simulink model "vehicleModelMotor"  (R2024b)
settings: Solver=VariableStepAuto  StartTime=0.0  StopTime=1200  MaxStep=0.1  RelTol=1e-3  AbsTol=1e-3
PreLoadFcn:
  | setVehicleParam
undefined symbols (not defined in the file): wheelInertia
libraries: fl_lib x8, sdl_lib x8, nesl_utility x5, ee_lib x3
settings Model: Creator=lnicolet  LastModifiedBy=lnicolet
settings SolverCC: AutoScaleAbsTol=off  AlgebraicLoopSolver=TrustRegion  MaxZcPerStep=1
settings DebuggingCC: UnconnectedInputMsg=warning  UnconnectedOutputMsg=warning  UnconnectedLineMsg=warning  SymbolicDimsDataTypeCodeGenerationDiagnostic=none
settings ModelReferenceCC: EnableRefExpFcnMdlSchedulingChecks=on
settings SFSimCC: CustomCodeUndefinedFunction=UseInterfaceOnly
settings RTWCC: GPUComputeCapability=3.5  DLArmComputeVersion=19.05
settings SimscapeCC: SimscapeLogType=all  SimscapeLogSimulationStatistics=on  SimscapeLogLimitData=off  SimscapeLogDataHistory=10000

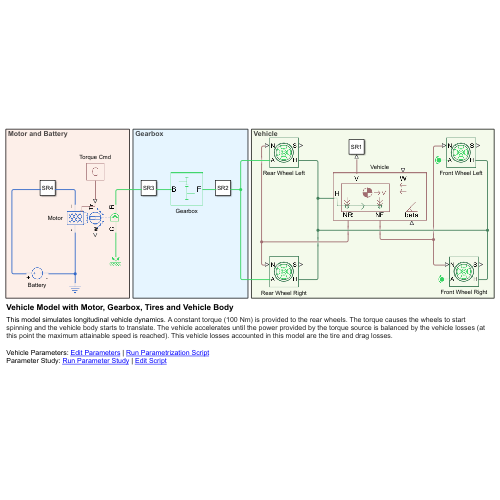
[thumbnail: Simulink's stored preview of the top-level diagram]
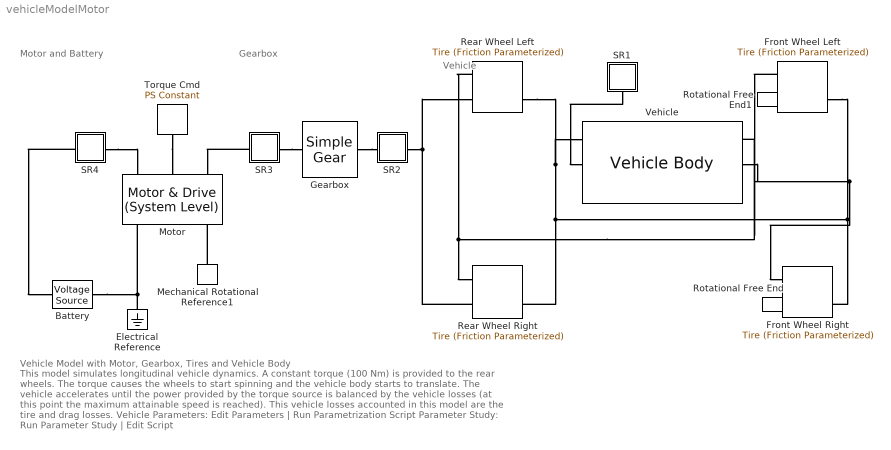
== system vehicleModelMotor ==
  note: Vehicle
  note: Gearbox
  note: This model simulates longitudinal vehicle dynamics. A constant torque (100 Nm) is provided to the rear wheels. The torque causes the wheels to start spinning and the vehicle body starts to translate. The vehicle accelerates until the power provided by the torque source is balanced by the vehicle losses (at this point the maximum attainable speed is reached). This vehicle losses accounted in this model are the tire and drag losses.
      |
      | Vehicle Parameters: Edit Parameters | Run Parametrization Script
      | Parameter Study: Run Parameter Study | Edit Script
  note: Vehicle Model with Motor, Gearbox, Tires and Vehicle Body
  note: Motor and Battery
  Battery : ee_lib/Sources/Voltage Source  dc_voltage=300 V  ac_voltage=0 V  ac_shift=0 rad  ac_frequency=60 Hz  noise_mode=ee.enum.sources.noise.Disabled  PSD=0 V^2/Hz  sample_time=1e-3 s  repeatability=ee.enum.sources.repeatability.NotRepeatable  user_seed=0  auto_seed=545404223  i_specify=off  i_priority=None  i=0 A  i_nominal_specify=off  i_nominal_value=1  i_nominal_unit=A  v_specify=off  v_priority=None  v=0 V  v_nominal_specify=off  v_nominal_value=1  v_nominal_unit=V
  Electrical Reference : fl_lib/Electrical/Electrical Elements/Electrical Reference
  Front Wheel Left : sdl_lib/Tires & Vehicles/Tire (Friction Parameterized)  r_tire=wheelRadius m  slip_output=sdl.enum.SlipOutput.Relative  friction_model=sdl.enum.friction_model_var.fixed  mu_static=0.90  mu_kinetic=0.70  slip_vector=[-1, .6, .15, .06, .02, 0] rad/s  mu_kinetic_vector=[.7, .7, .75, .8, .88, .89]  interp_method=simscape.enum.interpolation.linear  extrap_method=simscape.enum.extrapolation.linear  model_compliance=sdl.enum.compliance.off  stiffness=1e6 N/m  damping=1000 N*s/m  model_inertia=true  wheel_inertia=wheelInertia(1) kg*m^2  belt_inertia=wheelInertia(2) kg*m^2  initial_velocity=wheelSpeedStart rad/s  model_resistance=simscape.enum.onoff.on  resistance_model=sdl.enum.RollingResistance.Constant  coeff=0.015  p_tire=250e3 Pa  alpha=-0.003  beta=0.97  coeff_a=84e-4  coeff_b=6.2e-4 s/m  coeff_c=1.6e-4 s^2/m^2  v_thr=0.001 m/s  v_tol=0.001 m/s  F_min=10 N  initial_traction_state=sdl.enum.tireIC.slipping
      settings: InternalSimscapePortConfiguration="{\"Bottom\":[],\"Left\":[{\"id\":\"N\",\"label\":\"N\",\"type\":\"input\"},{\"id\":\"A\",\"label\":\"A\",\"type\":\"foundation.mechanical.rotational.rotational\"}],\"Right\":[{\"id\":\"Srel\",\"label\":\"S\",\"type\":\"output\"},{\"id\":\"H\",\"label\":\"H\",\"type\":\"foundation.mechanical.translational.translational\"}],\"Top\":[]}"
  Front Wheel Right : sdl_lib/Tires & Vehicles/Tire (Friction Parameterized)  r_tire=wheelRadius m  slip_output=sdl.enum.SlipOutput.Relative  friction_model=sdl.enum.friction_model_var.fixed  mu_static=0.90  mu_kinetic=0.70  slip_vector=[-1, .6, .15, .06, .02, 0] rad/s  mu_kinetic_vector=[.7, .7, .75, .8, .88, .89]  interp_method=simscape.enum.interpolation.linear  extrap_method=simscape.enum.extrapolation.linear  model_compliance=sdl.enum.compliance.off  stiffness=1e6 N/m  damping=1000 N*s/m  model_inertia=true  wheel_inertia=wheelInertia(1) kg*m^2  belt_inertia=wheelInertia(2) kg*m^2  initial_velocity=wheelSpeedStart rad/s  model_resistance=simscape.enum.onoff.on  resistance_model=sdl.enum.RollingResistance.Constant  coeff=0.015  p_tire=250e3 Pa  alpha=-0.003  beta=0.97  coeff_a=84e-4  coeff_b=6.2e-4 s/m  coeff_c=1.6e-4 s^2/m^2  v_thr=0.001 m/s  v_tol=0.001 m/s  F_min=10 N  initial_traction_state=sdl.enum.tireIC.slipping
      settings: InternalSimscapePortConfiguration="{\"Bottom\":[],\"Left\":[{\"id\":\"N\",\"label\":\"N\",\"type\":\"input\"},{\"id\":\"A\",\"label\":\"A\",\"type\":\"foundation.mechanical.rotational.rotational\"}],\"Right\":[{\"id\":\"Srel\",\"label\":\"S\",\"type\":\"output\"},{\"id\":\"H\",\"label\":\"H\",\"type\":\"foundation.mechanical.translational.translational\"}],\"Top\":[]}"
  Gearbox : sdl_lib/Gears/Simple Gear  ratio=gearboxRatio  rotation_direction=sdl.enum.shaftOutputDirection.same  friction_model=sdl.enum.gear_efficiencies_load.constant  T_noload=0.1 N*m  T_nom=5 N*m  efficiency_nom=0.8  efficiency=gearboxEff  temperature_TLU=[280, 300, 320] K  load_TLU=[1, 5, 10] N*m  efficiency_TLU=[.95, .9, .85]  efficiency_TLU2=[.85, .8, .75; .95, .9, .85; .85, .8, .7]  w_thr=0.01 rad/s  pwr_thr=0.001 W  enable_backlash=false  hardstop_model=simscape.enum.hardstop.smooth  backlash_distance=1e-3 mm  r_base=0.1 m  transition=1e-4 mm  backlash_stiffness=1e6 N/m  backlash_damping=1e3 N*s/m  coeff_rest=0.7  v_tol=0.001 m/s  f_tol=0.001 N  mu_visc=[0, 0] N*m*s/rad  thermal_mass=50 J/K  temperature_specify=off  temperature_priority=High  temperature=300 K  temperature_nominal_specify=off  temperature_nominal_value=1  temperature_nominal_unit=K  x_backlash_specify=off  x_backlash_priority=None  x_backlash=0 mm  x_backlash_nominal_specify=off  x_backlash_nominal_value=1  x_backlash_nominal_unit=mm  f_hardstop_specify=off  f_hardstop_priority=None  f_hardstop=0 N  f_hardstop_nominal_specify=off  f_hardstop_nominal_value=1  f_hardstop_nominal_unit=N  v_backlash_specify=off  v_backlash_priority=None  v_backlash=0 m/s  v_backlash_nominal_specify=off  v_backlash_nominal_value=1  v_backlash_nominal_unit=m/s
  Mechanical Rotational Reference1 : fl_lib/Mechanical/Rotational Elements/Mechanical Rotational Reference
  Motor : ee_lib/Electromechanical/Motor & Drive (System Level)  torque_speed_param=ee.enum.electromech.envelope.tabulated  overtorque_param=ee.enum.electromech.overtorque.no  T_t=EMTorque N*m  T_t_intermittent=[.36, .32, .28, 0] N*m  T_t_2D=[.09, .09, .09; .08, .08, .08; .07, .07, .07; 0, 0, 0] N*m  T_t_intermittent_2D=[.36, .36, .36; .32, .32, .32; .28, .28, .28; 0, 0, 0] N*m  w_t=EMSpeed rad/s  vdc_t=[6, 12, 24] V  torque_max=0.1 N*m  power_max=30 W  torque_max_intermittent=0.4 N*m  power_max_intermittent=120 W  time_overtorque=30 s  time_recover=60 s  Tc=0.02 s  EnableSwitch=false  losses_param=3  eff=100  w_eff=3750 rpm  T_eff=0.08 N*m  Piron=0 W  Pbase=0 W  w_eff_vec=EMSpeedEff rad/s  T_eff_vec=EMTorqueEff N*m  v_eff_vec=[100, 250, 400] V  losses_mat=[1.49, 1.67, 2.21, 3.1; .42, .69, 1.14, 2.03; .06, .24, .78, 1.68; .42, .69, 1.14, 2.03; 1.49, 1.67, 2.21, 3.1] W  efficiency_mat=EMEffMap  losses_mat_3D=ones(5, 4, 3) W  efficiency_mat_3D=95 * ones(5, 4, 3)  Res=0 Ohm  J=5e-6 kg*m^2  lam=1e-5 N*m*s/rad  speed0=0 rpm  fault_condition=1  fault_threshold=0.5  faulted_specify=off  faulted_priority=None  faulted=0  faulted_nominal_specify=off  faulted_nominal_value=1  faulted_nominal_unit=1  isSwitchedOff_specify=off  isSwitchedOff_priority=None  isSwitchedOff=0  isSwitchedOff_nominal_specify=off  isSwitchedOff_nominal_value=1  isSwitchedOff_nominal_unit=1  torqueLimitContinuous_specify=off  torqueLimitContinuous_priority=None  torqueLimitContinuous=0 N*m  torqueLimitContinuous_nominal_specify=off  torqueLimitContinuous_nominal_value=1  torqueLimitContinuous_nominal_unit=N*m  alpha=3.93e-3 1/K  Tmeas=25 degC  Tmeas2=125 degC  losses_mat_T2=[1.49, 1.74, 2.49, 3.74; .42, .67, 1.42, 2.67; .06, .31, 1.06, 2.31; .42, .67, 1.42, 2.67; 1.49, 1.74, 2.49, 3.74] W  efficiency_mat_T2=[95, 95, 95, 95; 95, 95, 95, 95; 95, 95, 95, 95; 95, 95, 95, 95; 95, 95, 95, 95]  losses_mat_3D_T2=ones(5, 4, 3) W  efficiency_mat_3D_T2=95 * ones(5, 4, 3)  thermal_mass=100 J/K  initial_temperature=25 degC
  Rear Wheel Left : sdl_lib/Tires & Vehicles/Tire (Friction Parameterized)  r_tire=wheelRadius m  slip_output=sdl.enum.SlipOutput.Relative  friction_model=sdl.enum.friction_model_var.fixed  mu_static=0.90  mu_kinetic=0.70  slip_vector=[-1, .6, .15, .06, .02, 0] rad/s  mu_kinetic_vector=[.7, .7, .75, .8, .88, .89]  interp_method=simscape.enum.interpolation.linear  extrap_method=simscape.enum.extrapolation.linear  model_compliance=sdl.enum.compliance.off  stiffness=1e6 N/m  damping=1000 N*s/m  model_inertia=true  wheel_inertia=wheelInertia(1) kg*m^2  belt_inertia=wheelInertia(2) kg*m^2  initial_velocity=wheelSpeedStart rad/s  model_resistance=simscape.enum.onoff.on  resistance_model=sdl.enum.RollingResistance.Constant  coeff=0.015  p_tire=250e3 Pa  alpha=-0.003  beta=0.97  coeff_a=84e-4  coeff_b=6.2e-4 s/m  coeff_c=1.6e-4 s^2/m^2  v_thr=0.001 m/s  v_tol=0.001 m/s  F_min=10 N  initial_traction_state=sdl.enum.tireIC.slipping
      settings: InternalSimscapePortConfiguration="{\"Bottom\":[],\"Left\":[{\"id\":\"N\",\"label\":\"N\",\"type\":\"input\"},{\"id\":\"A\",\"label\":\"A\",\"type\":\"foundation.mechanical.rotational.rotational\"}],\"Right\":[{\"id\":\"Srel\",\"label\":\"S\",\"type\":\"output\"},{\"id\":\"H\",\"label\":\"H\",\"type\":\"foundation.mechanical.translational.translational\"}],\"Top\":[]}"
  Rear Wheel Right : sdl_lib/Tires & Vehicles/Tire (Friction Parameterized)  r_tire=wheelRadius m  slip_output=sdl.enum.SlipOutput.Relative  friction_model=sdl.enum.friction_model_var.fixed  mu_static=0.90  mu_kinetic=0.70  slip_vector=[-1, .6, .15, .06, .02, 0] rad/s  mu_kinetic_vector=[.7, .7, .75, .8, .88, .89]  interp_method=simscape.enum.interpolation.linear  extrap_method=simscape.enum.extrapolation.linear  model_compliance=sdl.enum.compliance.off  stiffness=1e6 N/m  damping=1000 N*s/m  model_inertia=true  wheel_inertia=wheelInertia(1) kg*m^2  belt_inertia=wheelInertia(2) kg*m^2  initial_velocity=wheelSpeedStart rad/s  model_resistance=simscape.enum.onoff.on  resistance_model=sdl.enum.RollingResistance.Constant  coeff=0.015  p_tire=250e3 Pa  alpha=-0.003  beta=0.97  coeff_a=84e-4  coeff_b=6.2e-4 s/m  coeff_c=1.6e-4 s^2/m^2  v_thr=0.001 m/s  v_tol=0.001 m/s  F_min=10 N  initial_traction_state=sdl.enum.tireIC.slipping
      settings: InternalSimscapePortConfiguration="{\"Bottom\":[],\"Left\":[{\"id\":\"N\",\"label\":\"N\",\"type\":\"input\"},{\"id\":\"A\",\"label\":\"A\",\"type\":\"foundation.mechanical.rotational.rotational\"}],\"Right\":[{\"id\":\"Srel\",\"label\":\"S\",\"type\":\"output\"},{\"id\":\"H\",\"label\":\"H\",\"type\":\"foundation.mechanical.translational.translational\"}],\"Top\":[]}"
  Rotational Free End : fl_lib/Mechanical/Rotational Elements/Rotational Free End  w_specify=off  w_priority=None  w=0 rad/s  w_nominal_specify=off  w_nominal_value=1  w_nominal_unit=rad/s
  Rotational Free End1 : fl_lib/Mechanical/Rotational Elements/Rotational Free End  w_specify=off  w_priority=None  w=0 rad/s  w_nominal_specify=off  w_nominal_value=1  w_nominal_unit=rad/s
  SR1 : Subsystem
      settings: OpenFcn=|
      | scopePath = [gcb '/Scope'];
      | open_system(scopePath);
      mask Display: disp(get_param(gcb,'Name'));
  SR2 : Subsystem
      settings: PortSchema="{\"entries\":[{\"content\":{\"sides\":[{\"content\":{},\"type\":\"ConnectorPlacement.EquallySpacedRectSide\",\"uuid\":\"85a1558c-1b31-403a-adff-1ac0e6328287\"},{\"content\":{\"side\":\"RIGHT\"},\"type\":\"ConnectorPlacement.EquallySpacedRectSide\",\"uuid\":\"de598219-9a5a-4194-bdeb-930f1cdc45c3\"},{\"content\":{\"connectorIds\":[\"LConn1\"],\"side\":\"TOP\"},\"type\":\"ConnectorPlacement.EquallySpacedRectSide\",\"uuid\":\"10bc604a-047d-4d1a-b0b7-1fa83a2f0568\"},{\"content\":{\"connectorIds\":[\"RConn1\"],\"side\":\"BOTTOM\"},\"type\":\"ConnectorPlacement.EquallySpacedRectSide\",\"uuid\":\"148b1bdb-f9c4-471d-a1fa-71cb1ae939b1\"}]},\"type\":\"ConnectorPlacement.EquallySpacedConnector\",\"uuid\":\"121a5661-41e8-4645-ac4e-8b084eb01302\"}],\"packageUris\":[\"http://schema.mathworks.com/mf0/Connector/R2020b\"],\"version\":\"1.0\"}"
      settings: OpenFcn=|
      | scopePath = [gcb '/Scope'];
      | open_system(scopePath);
      mask Display: disp(get_param(gcb,'Name'))
  SR3 : Subsystem
      settings: PortSchema="{\"entries\":[{\"content\":{\"sides\":[{\"content\":{},\"type\":\"ConnectorPlacement.EquallySpacedRectSide\",\"uuid\":\"85a1558c-1b31-403a-adff-1ac0e6328287\"},{\"content\":{\"side\":\"RIGHT\"},\"type\":\"ConnectorPlacement.EquallySpacedRectSide\",\"uuid\":\"de598219-9a5a-4194-bdeb-930f1cdc45c3\"},{\"content\":{\"connectorIds\":[\"LConn1\"],\"side\":\"TOP\"},\"type\":\"ConnectorPlacement.EquallySpacedRectSide\",\"uuid\":\"10bc604a-047d-4d1a-b0b7-1fa83a2f0568\"},{\"content\":{\"connectorIds\":[\"RConn1\"],\"side\":\"BOTTOM\"},\"type\":\"ConnectorPlacement.EquallySpacedRectSide\",\"uuid\":\"148b1bdb-f9c4-471d-a1fa-71cb1ae939b1\"}]},\"type\":\"ConnectorPlacement.EquallySpacedConnector\",\"uuid\":\"121a5661-41e8-4645-ac4e-8b084eb01302\"}],\"packageUris\":[\"http://schema.mathworks.com/mf0/Connector/R2020b\"],\"version\":\"1.0\"}"
      settings: OpenFcn=|
      | scopePath = [gcb '/Scope'];
      | open_system(scopePath);
      mask Display: disp(get_param(gcb,'Name'))
  SR4 : Subsystem
      settings: PortSchema="{\"entries\":[{\"content\":{\"sides\":[{\"content\":{},\"type\":\"ConnectorPlacement.EquallySpacedRectSide\",\"uuid\":\"85a1558c-1b31-403a-adff-1ac0e6328287\"},{\"content\":{\"side\":\"RIGHT\"},\"type\":\"ConnectorPlacement.EquallySpacedRectSide\",\"uuid\":\"de598219-9a5a-4194-bdeb-930f1cdc45c3\"},{\"content\":{\"connectorIds\":[\"LConn1\"],\"side\":\"TOP\"},\"type\":\"ConnectorPlacement.EquallySpacedRectSide\",\"uuid\":\"10bc604a-047d-4d1a-b0b7-1fa83a2f0568\"},{\"content\":{\"connectorIds\":[\"RConn1\"],\"side\":\"BOTTOM\"},\"type\":\"ConnectorPlacement.EquallySpacedRectSide\",\"uuid\":\"148b1bdb-f9c4-471d-a1fa-71cb1ae939b1\"}]},\"type\":\"ConnectorPlacement.EquallySpacedConnector\",\"uuid\":\"121a5661-41e8-4645-ac4e-8b084eb01302\"}],\"packageUris\":[\"http://schema.mathworks.com/mf0/Connector/R2020b\"],\"version\":\"1.0\"}"
      settings: OpenFcn=|
      | scopePath = [gcb '/Scope'];
      | open_system(scopePath);
      mask Display: disp(get_param(gcb,'Name'))
  Torque Cmd : fl_lib/Physical Signals/Sources/PS Constant  constant=100 N*m
  Vehicle : sdl_lib/Tires & Vehicles/Vehicle Body  mass=vehicleMass kg  n_w=2  x_f=vehicleCOGFA m  x_r=vehicleCOGRA m  y_c=0.5 m  mass_var=false  g=9.81 m/s^2  liftoff_warning=false  area=vehicleSurf m^2  Cd_var=false  Cd=vehicleCD  rho=1.18 kg/m^3  model_pitch=false  inertia=4000 kg*m^2  suspension_model=sdl.enum.linearTLU.linear  k_f=1e4 N/m  b_f=1e4 N*s/m  k_r=1e4 N/m  b_r=1e4 N*s/m  k_f_TLU=[-2000, -1000, 0, 1000, 2000] N  x_f_TLU=[-.4, -.2, 0, .2, .4] m  b_f_TLU=[-200, -100, 0, 100, 200] N  v_f_TLU=[-4, -2, 0, 2, 4] m/s  k_r_TLU=[-2000, -1000, 0, 1000, 2000] N  x_r_TLU=[-.4, -.2, 0, .2, .4] m  b_r_TLU=[-200, -100, 0, 100, 200] N  v_r_TLU=[-4, -2, 0, 2, 4] m/s  interp_method=simscape.enum.interpolation.linear  extrap_method=simscape.enum.extrapolation.linear  model_hardstop=false  upper_bound_f=.25 m  lower_bound_f=-.25 m  stop_k_f=1e6 N/m  stop_b_f=150 N*s/m  upper_bound_r=.25 m  lower_bound_r=-.25 m  stop_k_r=1e6 N/m  stop_b_r=150 N*s/m  initial_pitch=0 rad  initial_pitch_rate=0 rad/s  v_specify=on  v_priority=High  v=0 m/s  v_nominal_specify=off  v_nominal_value=1  v_nominal_unit=m/s
      settings: InternalSimscapePortConfiguration="{\"Bottom\":[{\"id\":\"NR\",\"label\":\"NR\",\"type\":\"output\"},{\"id\":\"NF\",\"label\":\"NF\",\"type\":\"output\"},{\"id\":\"beta\",\"label\":\"beta\",\"type\":\"input\"}],\"Left\":[{\"id\":\"H\",\"label\":\"H\",\"type\":\"foundation.mechanical.translational.translational\"}],\"Right\":[],\"Top\":[{\"id\":\"V\",\"label\":\"V\",\"type\":\"output\"},{\"id\":\"wind\",\"label\":\"W\",\"type\":\"input\"}]}"
  connections:
  Rear Wheel Left/RConn2 -- Rear Wheel Right/RConn2 -- Front Wheel Right/RConn2 -- Front Wheel Left/RConn2 -- Vehicle/LConn1
  Rear Wheel Left/LConn1 -- Rear Wheel Right/LConn1 -- Vehicle/RConn1
  Vehicle/RConn2 -- Front Wheel Left/LConn1 -- Front Wheel Right/LConn1
  SR1/LConn1 -- Vehicle/LConn2
  Rear Wheel Right/LConn2 -- Rear Wheel Left/LConn2 -- SR2/RConn1
  Rotational Free End/LConn1 -- Front Wheel Right/LConn2
  Rotational Free End1/LConn1 -- Front Wheel Left/LConn2
  Gearbox/RConn1 -- SR2/LConn1
  SR3/RConn1 -- Gearbox/LConn1
  SR3/LConn1 -- Motor/LConn3
  Torque Cmd/RConn1 -- Motor/LConn2
  Mechanical Rotational Reference1/LConn1 -- Motor/RConn3
  Battery/RConn1 -- Motor/RConn1 -- Electrical Reference/LConn1
  SR4/RConn1 -- Motor/LConn1
  SR4/LConn1 -- Battery/LConn1

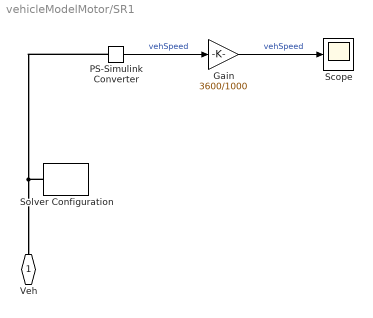
== system vehicleModelMotor/SR1 ==
  Gain : Gain  Gain=3600/1000
  PS-Simulink Converter : nesl_utility/PS-Simulink Converter  PhysicalDomain=network_engine_domain  SubClassName=ps_output  LeftPortType=input  RightPortType=output  PseudoPeriodic=off  Frequencies=[]  VectorFormat=inherit  Unit=m/s  AffineConversion=off
  Scope : Scope
  Solver Configuration : nesl_utility/Solver Configuration  PhysicalDomain=network_engine_domain  SubClassName=solver  LeftPortType=input  RightPortType=generic  Tones=[]  Harmonics=[]  SimulateNoise=off  Profile=off  UseLocalSampling=off  EnableSwitchedLinearOptims=on  FrequencyDomain=off  UseCCode=off  RelTol=0.001  AbsTol=1e-06  MinStep=1e-09  ToWorkspace=off  RevertToSquareIcSolve=off  NumHomotopyIterations=100  PhasorMode=off  PhasorModeNumHarmonics=1  ConsistencySolver=NEWTON_XTOL_AFTER_FTOL  IndexReductionMethod=DerivativeReplacement  DoDC=off  ResidualTolerance=1e-09  ConsistencyTolSource=GLOBAL  ConsistencyAbsTol=0.001  ConsistencyRelTol=0.001  ConsistencyTolFactor=0.001  UseLocalSolver=off  LocalSolverChoice=NE_BACKWARD_EULER_ADVANCER  ResolveIndetEquations=on  FunctionEvalNumThread=1  LocalSolverSampleTime=0.001  DoFixedCost=off  MaxNonlinIter=3  MaxModeIter=2  ComputeImpulses=off  ImpulseIterations=2  LinearAlgebra=auto  LinearAlgebraNumThread=0  EquationFormulation=NE_TIME_EF  DelaysMemoryBudget=1024  AutomaticFiltering=on  FilteringTimeConstant=0.001  PartitionStorageMethod=AS_NEEDED  PartitionMemoryBudget=1024  PartitionMethod=ROBUST  MultibodyUseLocalSolver=off  MultibodyLocalSolverChoice=ODE1  MultibodyLocalSolverSampleTime=0.001
  Veh : PMIOPort  Side=Left
  wires:
  PS-Simulink Converter/1 -> Gain/1  "vehSpeed"
  Gain/1 -> Scope/1  "vehSpeed"
  connections:
  PS-Simulink Converter/LConn1 -- Veh/RConn1 -- Solver Configuration/RConn1

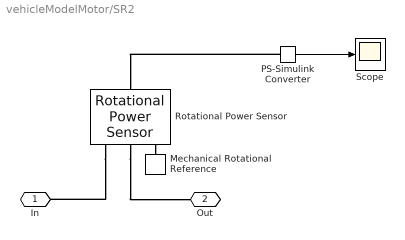
== system vehicleModelMotor/SR2 ==
  Mechanical Rotational Reference : fl_lib/Mechanical/Rotational Elements/Mechanical Rotational Reference
  PS-Simulink Converter : nesl_utility/PS-Simulink Converter  PhysicalDomain=network_engine_domain  SubClassName=ps_output  LeftPortType=input  RightPortType=output  PseudoPeriodic=off  Frequencies=[]  VectorFormat=inherit  Unit=kW  AffineConversion=off
  Rotational Power Sensor : sdl_lib/Sensors/Rotational Power Sensor  measurement_type=sdl.enum.rotationalPowerSensorType.instantaneous  averaging_period=1 s  max_frequency=1000 Hz  max_speed=1000 rpm
      settings: InternalSimscapePortConfiguration="{\"Bottom\":[],\"Left\":[{\"id\":\"S\",\"label\":\"S\",\"type\":\"foundation.mechanical.rotational.rotational\"},{\"id\":\"R\",\"label\":\"R\",\"type\":\"foundation.mechanical.rotational.rotational\"},{\"id\":\"C\",\"label\":\"C\",\"type\":\"foundation.mechanical.rotational.rotational\"}],\"Right\":[{\"id\":\"P\",\"label\":\"P\",\"type\":\"output\"}],\"Top\":[]}"
  Scope : Scope
  In : PMIOPort  Side=Left
  Out : PMIOPort  Port=2  Side=Right
  wires:
  PS-Simulink Converter/1 -> Scope/1
  connections:
  Rotational Power Sensor/LConn1 -- In/RConn1
  Rotational Power Sensor/LConn2 -- Out/RConn1
  Rotational Power Sensor/LConn3 -- Mechanical Rotational Reference/LConn1
  PS-Simulink Converter/LConn1 -- Rotational Power Sensor/RConn1

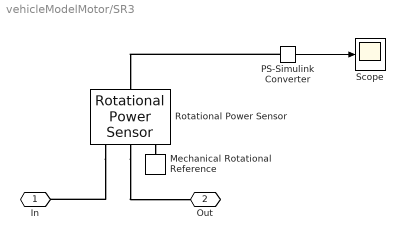
== system vehicleModelMotor/SR3 ==
  Mechanical Rotational Reference : fl_lib/Mechanical/Rotational Elements/Mechanical Rotational Reference
  PS-Simulink Converter : nesl_utility/PS-Simulink Converter  PhysicalDomain=network_engine_domain  SubClassName=ps_output  LeftPortType=input  RightPortType=output  PseudoPeriodic=off  Frequencies=[]  VectorFormat=inherit  Unit=kW  AffineConversion=off
  Rotational Power Sensor : sdl_lib/Sensors/Rotational Power Sensor  measurement_type=sdl.enum.rotationalPowerSensorType.instantaneous  averaging_period=1 s  max_frequency=1000 Hz  max_speed=1000 rpm
      settings: InternalSimscapePortConfiguration="{\"Bottom\":[],\"Left\":[{\"id\":\"S\",\"label\":\"S\",\"type\":\"foundation.mechanical.rotational.rotational\"},{\"id\":\"R\",\"label\":\"R\",\"type\":\"foundation.mechanical.rotational.rotational\"},{\"id\":\"C\",\"label\":\"C\",\"type\":\"foundation.mechanical.rotational.rotational\"}],\"Right\":[{\"id\":\"P\",\"label\":\"P\",\"type\":\"output\"}],\"Top\":[]}"
  Scope : Scope
  In : PMIOPort  Side=Left
  Out : PMIOPort  Port=2  Side=Right
  wires:
  PS-Simulink Converter/1 -> Scope/1
  connections:
  Rotational Power Sensor/LConn1 -- In/RConn1
  Rotational Power Sensor/LConn2 -- Out/RConn1
  Rotational Power Sensor/LConn3 -- Mechanical Rotational Reference/LConn1
  PS-Simulink Converter/LConn1 -- Rotational Power Sensor/RConn1

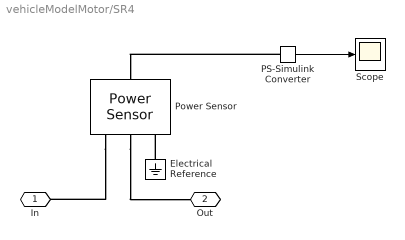
== system vehicleModelMotor/SR4 ==
  Electrical Reference : fl_lib/Electrical/Electrical Elements/Electrical Reference
  PS-Simulink Converter : nesl_utility/PS-Simulink Converter  PhysicalDomain=network_engine_domain  SubClassName=ps_output  LeftPortType=input  RightPortType=output  PseudoPeriodic=off  Frequencies=[]  VectorFormat=inherit  Unit=kW  AffineConversion=off
  Power Sensor : ee_lib/Sensors & Transducers/Power Sensor  measurement_type=1  averaging_period=1e-4 s
  Scope : Scope
  In : PMIOPort  Side=Left
  Out : PMIOPort  Port=2  Side=Right
  wires:
  PS-Simulink Converter/1 -> Scope/1
  connections:
  Power Sensor/LConn1 -- In/RConn1
  Power Sensor/LConn2 -- Out/RConn1
  PS-Simulink Converter/LConn1 -- Power Sensor/RConn1
  Electrical Reference/LConn1 -- Power Sensor/LConn3
